simulink model "sim_2_twolink_joint_control_real"  (R2021a)
settings: Solver=ode45  StartTime=0.0  StopTime=15  MaxStep=0.01  RelTol=1e-5  EnableMultiTasking=on
values from neighbouring files (symbols this model uses):
  b1 = 0.01    [sim_params.m]    (also in sim_params_force.m)
  b2 = 0.01    [sim_params.m]    (also in sim_params_force.m)
  D = [zeros(n); eye(n)]    [control_comparison_script.m]    (also in gen_twolink_ss.m = reshape([0.0,0.0,0.0,0.0,0.0,0.0,0.0,0.0],[4,2]))
  D_T_Q = D'*Q    [control_comparison_script.m]
  epsilon = 0.1    [control_comparison_script.m]
  g = 9.80665    [sim_params.m]    (also in sim_params_force.m)
  joint_acc_variance = 0    [sim_params.m]    (also in sim_params_force.m)
  joint_pos_variance = joint_pos_precision^2    (= 0.0001)    [control_comparison_script.m]    (also in sim_params.m = 2.5e-05; sim_params_force.m = 2.5e-05)
  joint_vel_variance = 0    [sim_params.m]    (also in sim_params_force.m)
  Kd1 = 2.5    [control_comparison_script.m]
  Kd1_grav = 2.5    [control_comparison_script.m]
  Kd1_inv = 12    [control_comparison_script.m]
  Kd1_robust = 7    [control_comparison_script.m]
  Kd2 = 0.5    [control_comparison_script.m]
  Kd2_grav = 0.5    [control_comparison_script.m]
  Kd2_inv = 15    [control_comparison_script.m]
  Kd2_robust = 35    [control_comparison_script.m]
  Ki1 = 20    [control_comparison_script.m]
  Ki2 = 15    [control_comparison_script.m]
  Klqr = lqr(A,B,Q,R)    [control_comparison_script.m]
  Kp1 = 30    [control_comparison_script.m]
  Kp1_grav = 15    [control_comparison_script.m]
  Kp1_inv = 25    [control_comparison_script.m]
  Kp1_robust = 25    [control_comparison_script.m]
  Kp2 = 7    [control_comparison_script.m]
  Kp2_grav = 3.5    [control_comparison_script.m]
  Kp2_inv = 50    [control_comparison_script.m]
  Kp2_robust = 45    [control_comparison_script.m]
  Kpp = place(A,B,p)    [control_comparison_script.m]
  L1x = 0.3    [sim_params.m]    (also in sim_params_force.m)
  L1y = 0.050    (= 0.05)    [sim_params.m]    (also in sim_params_force.m)
  L1z = 0.05    [sim_params.m]    (also in sim_params_force.m)
  L2x = 0.15    [sim_params.m]    (also in sim_params_force.m = 0.3)
  L2y = 0.05    [sim_params.m]    (also in sim_params_force.m)
  L2z = 0.05    [sim_params.m]    (also in sim_params_force.m)
  length_dev = (100+randi([-param_dev,param_dev],1))/100.0    [control_comparison_script.m]
  m1 = m1*1.25    [control_comparison_script.m]    (also in sim_params.m = 2.775; sim_params_force.m = 2.775)
  m2 = m2*1.25    [control_comparison_script.m]    (also in sim_params.m = 1.3875; sim_params_force.m = 2.775)
  m_dev = (100+randi([-param_dev,param_dev],1))/100.0    [control_comparison_script.m]
  max_joint_torque1 = 20    [sim_params.m]    (also in sim_params_force.m)
  max_joint_torque2 = 10    [sim_params.m]    (also in sim_params_force.m = 20)
  N1 = 100    [control_comparison_script.m]
  N1_grav = 100    [control_comparison_script.m]
  N1_inv = 50    [control_comparison_script.m]
  N1_robust = 50    [control_comparison_script.m]
  N2 = 100    [control_comparison_script.m]
  N2_grav = 100    [control_comparison_script.m]
  N2_inv = 50    [control_comparison_script.m]
  N2_robust = 50    [control_comparison_script.m]
  rho = [1;1]    [control_comparison_script.m]
  theta1_0 = 0    [sim_params.m]    (also in sim_params_force.m = 1.57079632679)
  theta1_dot_0 = 0    [sim_params.m]    (also in sim_params_force.m)
  theta2_0 = 0    [sim_params.m]    (also in sim_params_force.m = -1.57079632679)
  theta2_dot_0 = 0    [sim_params.m]    (also in sim_params_force.m)
  Tsample = 0.001    [sim_params.m]    (also in sim_params_force.m)
  vis_dev = (100+randi([-param_dev,param_dev],1))/100.0    [control_comparison_script.m]
undefined symbols (not defined in the file or in its folder): gs, Ksm, phi_sm, sigbuilder_block, X, Y, Z
libraries: pid_lib x18, sm_lib x11, spsFirstOrderFilterLib x10, simulink_extras x10, nesl_utility x10, dspmtrx3 x2
(part 4 of 4)

== system sim_2_twolink_joint_control_real/Torqu limit/no-limit ==
  In1 : Inport
  Out1 : Outport
  wires:
  In1/1 -> Out1/1

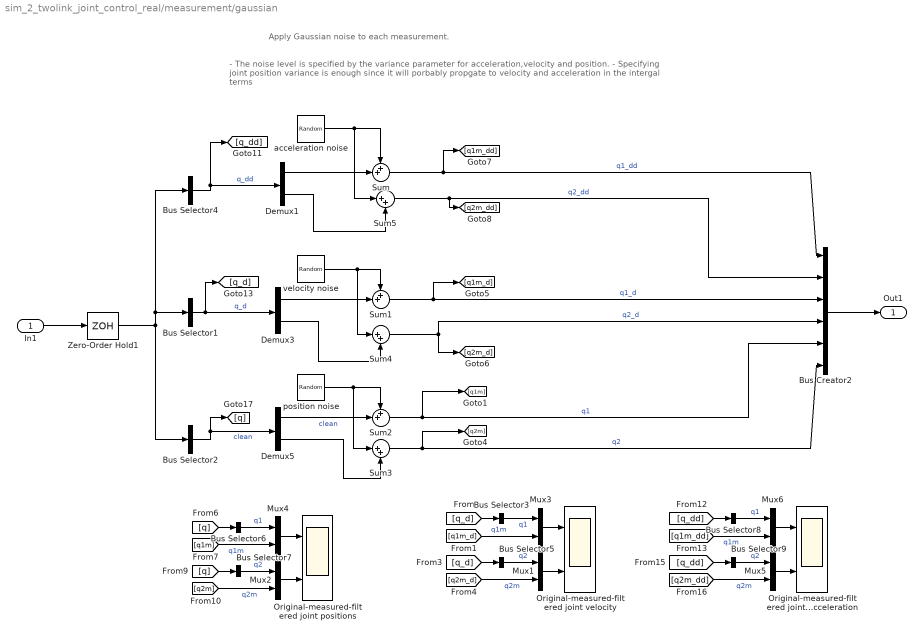
== system sim_2_twolink_joint_control_real/measurement/gaussian ==
  note: - The noise level is specified by the variance parameter for acceleration,velocity and position.
      | - Specifying joint position variance is enough since it will porbably propgate to velocity and acceleration in the intergal terms
  note: Apply Gaussian noise to each measurement.
  In1 : Inport
  Bus Creator2 : BusCreator  Inputs=6
  Bus Selector1 : BusSelector  OutputSignals=q1_d,q2_d  OutputAsBus=on
  Bus Selector2 : BusSelector  OutputSignals=q1,q2  OutputAsBus=on
  Bus Selector3 : BusSelector  OutputSignals=q1_d  OutputAsBus=on
  Bus Selector4 : BusSelector  OutputSignals=q1_dd,q2_dd  OutputAsBus=on
  Bus Selector5 : BusSelector  OutputSignals=q2_d  OutputAsBus=on
  Bus Selector6 : BusSelector  OutputSignals=q1  OutputAsBus=on
  Bus Selector7 : BusSelector  OutputSignals=q2  OutputAsBus=on
  Bus Selector8 : BusSelector  OutputSignals=q1_dd  OutputAsBus=on
  Bus Selector9 : BusSelector  OutputSignals=q2_dd  OutputAsBus=on
  Demux1 : Demux  Outputs=2
  Demux3 : Demux  Outputs=2
  Demux5 : Demux  Outputs=2
  Mux{1..6} (6 alike) : Mux  Inputs=2
  Original-measured-filtered joint Acceleration : Scope  NumInputPorts=2
  Original-measured-filtered joint positions : Scope  NumInputPorts=2
  Original-measured-filtered joint velocity : Scope  NumInputPorts=2
  Sum : Sum  Inputs=++|
  Sum1 : Sum  Inputs=++|
  Sum2 : Sum  Inputs=++|
  Sum3 : Sum  Inputs=|++
  Sum4 : Sum  Inputs=|++
  Sum5 : Sum  Inputs=|++
  Zero-Order Hold1 : ZeroOrderHold  SampleTime=Tsample
  acceleration noise : RandomNumber  Variance=joint_acc_variance  SampleTime=Tsample
  position noise : RandomNumber  Variance=joint_pos_variance  SampleTime=Tsample
  velocity noise : RandomNumber  Variance=joint_vel_variance  SampleTime=Tsample
  Out1 : Outport
  wires:
  In1/1 -> Zero-Order Hold1/1
  Demux1/1 -> Sum/2
  Demux3/2 -> Sum4/2
  Bus Selector3/1 -> Mux3/1  "q1"
  Mux2/1 -> Original-measured-filtered joint positions/2
  [q] -> Bus Selector6/1
  Bus Selector7/1 -> Mux2/1  "q2"
  [q1m] -> Mux4/2  "q1m"
  [q] -> Bus Selector7/1
  Bus Selector6/1 -> Mux4/1  "q1"
  Sum5/1 -> Bus Creator2/2, [q2m_dd]  "q2_dd"
  [q1m_d] -> Mux3/2  "q1m"
  Bus Selector4/1 -> [q_dd], Demux1/1  "q_dd"
  position noise/1 -> Sum2/1, Sum3/1
  Mux4/1 -> Original-measured-filtered joint positions/1
  velocity noise/1 -> Sum1/1, Sum4/1
  [q2m] -> Mux2/2  "q2m"
  Zero-Order Hold1/1 -> Bus Selector4/1, Bus Selector1/1, Bus Selector2/1
  Sum1/1 -> Bus Creator2/3, [q1m_d]  "q1_d"
  Mux5/1 -> Original-measured-filtered joint Acceleration/2
  Demux1/2 -> Sum5/2
  ? -> ?  "q2f"
  [q2m_dd] -> Mux5/2  "q2m"
  Bus Selector9/1 -> Mux5/1  "q2"
  [q_dd] -> Bus Selector8/1
  Sum2/1 -> Bus Creator2/5, [q1m]  "q1"
  acceleration noise/1 -> Sum5/1, Sum/1
  [q1m_dd] -> Mux6/2  "q1m"
  Bus Selector2/1 -> Demux5/1, [q]  "clean"
  Bus Creator2/1 -> Out1/1
  Bus Selector8/1 -> Mux6/1  "q1"
  [q_dd] -> Bus Selector9/1
  Mux6/1 -> Original-measured-filtered joint Acceleration/1
  Mux3/1 -> Original-measured-filtered joint velocity/1
  [q_d] -> Bus Selector3/1
  Demux5/1 -> Sum2/2  "clean"
  Demux5/2 -> Sum3/2
  Bus Selector5/1 -> Mux1/1  "q2"
  [q_d] -> Bus Selector5/1
  Bus Selector1/1 -> [q_d], Demux3/1  "q_d"
  Sum3/1 -> Bus Creator2/6, [q2m]  "q2"
  Sum/1 -> Bus Creator2/1, [q1m_dd]  "q1_dd"
  Sum4/1 -> Bus Creator2/4, [q2m_d]  "q2_d"
  [q2m_d] -> Mux1/2  "q2m"
  Demux3/1 -> Sum1/2
  Mux1/1 -> Original-measured-filtered joint velocity/2

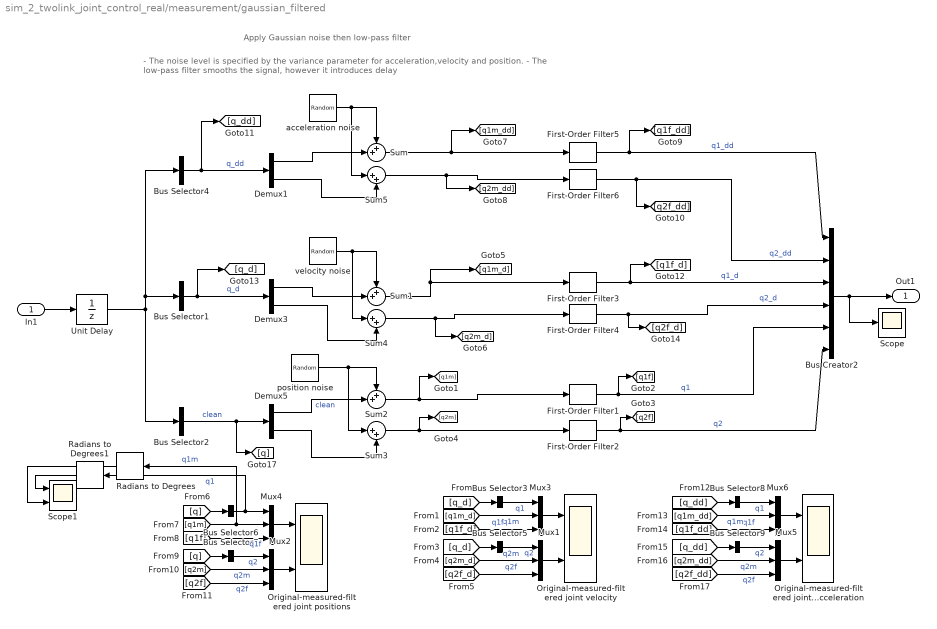
== system sim_2_twolink_joint_control_real/measurement/gaussian_filtered ==
  note: - The noise level is specified by the variance parameter for acceleration,velocity and position.
      | - The low-pass filter smooths the signal, however it introduces delay
  note: Apply Gaussian noise then low-pass filter
  In1 : Inport
  Bus Creator2 : BusCreator  Inputs=6
  Bus Selector1 : BusSelector  OutputSignals=q1_d,q2_d  OutputAsBus=on
  Bus Selector2 : BusSelector  OutputSignals=q1,q2  OutputAsBus=on
  Bus Selector3 : BusSelector  OutputSignals=q1_d  OutputAsBus=on
  Bus Selector4 : BusSelector  OutputSignals=q1_dd,q2_dd  OutputAsBus=on
  Bus Selector5 : BusSelector  OutputSignals=q2_d  OutputAsBus=on
  Bus Selector6 : BusSelector  OutputSignals=q1  OutputAsBus=on
  Bus Selector7 : BusSelector  OutputSignals=q2  OutputAsBus=on
  Bus Selector8 : BusSelector  OutputSignals=q1_dd  OutputAsBus=on
  Bus Selector9 : BusSelector  OutputSignals=q2_dd  OutputAsBus=on
  Demux1 : Demux  Outputs=2
  Demux3 : Demux  Outputs=2
  Demux5 : Demux  Outputs=2
  First-Order Filter1 : spsFirstOrderFilterLib/First-Order Filter  FilterType=Lowpass  Tc=0.006  Ts=Tsample  Initialize=on  Vac_Init=[0, 0, 0]  Vdc_Init=0  PlotResponse=off  FreqRange="[0,  200,  1]"
  First-Order Filter2 : spsFirstOrderFilterLib/First-Order Filter  FilterType=Lowpass  Tc=0.006  Ts=Tsample  Initialize=on  Vac_Init=[0, 0, 0]  Vdc_Init=0  PlotResponse=off  FreqRange="[0,  200,  1]"
  First-Order Filter3 : spsFirstOrderFilterLib/First-Order Filter  FilterType=Lowpass  Tc=0.05  Ts=Tsample  Initialize=on  Vac_Init=[0, 0, 0]  Vdc_Init=0  PlotResponse=off  FreqRange="[0,  200,  1]"
  First-Order Filter4 : spsFirstOrderFilterLib/First-Order Filter  FilterType=Lowpass  Tc=0.05  Ts=Tsample  Initialize=on  Vac_Init=[0, 0, 0]  Vdc_Init=0  PlotResponse=off  FreqRange="[0,  200,  1]"
  First-Order Filter5 : spsFirstOrderFilterLib/First-Order Filter  FilterType=Lowpass  Tc=0.1  Ts=Tsample  Initialize=on  Vac_Init=[0, 0, 0]  Vdc_Init=0  PlotResponse=off  FreqRange="[0,  200,  1]"
  First-Order Filter6 : spsFirstOrderFilterLib/First-Order Filter  FilterType=Lowpass  Tc=0.1  Ts=Tsample  Initialize=on  Vac_Init=[0, 0, 0]  Vdc_Init=0  PlotResponse=off  FreqRange="[0,  200,  1]"
  Mux{1..6} (6 alike) : Mux  Inputs=3
  Original-measured-filtered joint Acceleration : Scope  NumInputPorts=2
  Original-measured-filtered joint positions : Scope  NumInputPorts=2
  Original-measured-filtered joint velocity : Scope  NumInputPorts=2
  Radians to Degrees : simulink_extras/Transformations/Radians to Degrees
  Radians to Degrees1 : simulink_extras/Transformations/Radians to Degrees
  Scope : Scope
  Scope1 : Scope  NumInputPorts=2
  Sum : Sum  Inputs=++|
  Sum1 : Sum  Inputs=++|
  Sum2 : Sum  Inputs=++|
  Sum3 : Sum  Inputs=|++
  Sum4 : Sum  Inputs=|++
  Sum5 : Sum  Inputs=|++
  Unit Delay : UnitDelay  SampleTime=Tsample  HasFrameUpgradeWarning=on
  acceleration noise : RandomNumber  Variance=joint_acc_variance  SampleTime=Tsample
  position noise : RandomNumber  Variance=joint_pos_variance  SampleTime=Tsample
  velocity noise : RandomNumber  Variance=joint_vel_variance  SampleTime=Tsample
  Out1 : Outport
  wires:
  acceleration noise/1 -> Sum/1, Sum5/1
  Bus Selector4/1 -> [q_dd], Demux1/1  "q_dd"
  Sum4/1 -> First-Order Filter4/1, [q2m_d]
  velocity noise/1 -> Sum1/1, Sum4/1
  Demux3/1 -> Sum1/2
  Bus Selector1/1 -> [q_d], Demux3/1  "q_d"
  Sum2/1 -> [q1m], First-Order Filter1/1
  position noise/1 -> Sum2/1, Sum3/1
  Demux5/1 -> Sum2/2  "clean"
  In1/1 -> Unit Delay/1
  Bus Creator2/1 -> Scope/1, Out1/1
  First-Order Filter2/1 -> Bus Creator2/6, [q2f]  "q2"
  First-Order Filter1/1 -> Bus Creator2/5, [q1f]  "q1"
  First-Order Filter3/1 -> Bus Creator2/3, [q1f_d]  "q1_d"
  First-Order Filter4/1 -> Bus Creator2/4, [q2f_d]  "q2_d"
  First-Order Filter6/1 -> Bus Creator2/2, [q2f_dd]  "q2_dd"
  [q_d] -> Bus Selector3/1
  Mux3/1 -> Original-measured-filtered joint velocity/1
  Bus Selector3/1 -> Mux3/1  "q1"
  Bus Selector2/1 -> [q], Demux5/1  "clean"
  Demux5/2 -> Sum3/2
  Sum3/1 -> [q2m], First-Order Filter2/1
  [q1m_d] -> Mux3/2  "q1m"
  [q1f_d] -> Mux3/3  "q1f"
  [q2m_d] -> Mux1/2  "q2m"
  Mux1/1 -> Original-measured-filtered joint velocity/2
  [q2f_d] -> Mux1/3  "q2f"
  Bus Selector5/1 -> Mux1/1  "q2"
  [q_d] -> Bus Selector5/1
  Demux3/2 -> Sum4/2
  Sum1/1 -> First-Order Filter3/1, [q1m_d]
  Demux1/1 -> Sum/2
  Demux1/2 -> Sum5/2
  Sum/1 -> [q1m_dd], First-Order Filter5/1
  Sum5/1 -> [q2m_dd], First-Order Filter6/1
  Bus Selector6/1 -> Radians to Degrees1/1, Mux4/1  "q1"
  [q1f] -> Mux4/3  "q1f"
  [q1m] -> Radians to Degrees/1, Mux4/2  "q1m"
  Mux4/1 -> Original-measured-filtered joint positions/1
  Bus Selector7/1 -> Mux2/1  "q2"
  [q] -> Bus Selector7/1
  [q2m] -> Mux2/2  "q2m"
  [q] -> Bus Selector6/1
  Mux2/1 -> Original-measured-filtered joint positions/2
  [q2f] -> Mux2/3  "q2f"
  Bus Selector8/1 -> Mux6/1  "q1"
  [q1f_dd] -> Mux6/3  "q1f"
  [q1m_dd] -> Mux6/2  "q1m"
  Mux6/1 -> Original-measured-filtered joint Acceleration/1
  Bus Selector9/1 -> Mux5/1  "q2"
  [q_dd] -> Bus Selector9/1
  [q2m_dd] -> Mux5/2  "q2m"
  [q_dd] -> Bus Selector8/1
  Mux5/1 -> Original-measured-filtered joint Acceleration/2
  [q2f_dd] -> Mux5/3  "q2f"
  First-Order Filter5/1 -> Bus Creator2/1, [q1f_dd]  "q1_dd"
  Unit Delay/1 -> Bus Selector4/1, Bus Selector1/1, Bus Selector2/1
  Radians to Degrees1/1 -> Scope1/1
  Radians to Degrees/1 -> Scope1/2

== system sim_2_twolink_joint_control_real/measurement/ideal ==
  In1 : Inport
  Zero-Order Hold1 : ZeroOrderHold  SampleTime=Tsample
  Out1 : Outport
  wires:
  In1/1 -> Zero-Order Hold1/1
  Zero-Order Hold1/1 -> Out1/1

== system sim_2_twolink_joint_control_real/Commands/Step command/Joint commands ==
  Demux : Demux  Tag=STV Demux  Outputs=2
      settings: DisplayOption=none
  FromWs : FromWorkspace  Tag=STV FromWs  VariableName=tuvar
      SigBuilderData=|
      | common.afterFinalStr = 'Extrapolate'
      | common.sampleTime = 0
      | dataSet(1).timeRange = [0 1000]
      | dataSet(1).name = 'PULSES_SMALL'
      | dataSet(2).timeRange = [0 1000]
      | dataSet(2).name = 'ZERO'
      | dataSet(3).timeRange = [0 1000]
      | dataSet(3).name = 'PULSES_BIG'
      | dataSet(4).timeRange = [0 1000]
      | dataSet(4).name = 'PULSES_SMALL1'
      | sbobj.Groups(1).Name = 'PULSES_SMALL'
      | sbobj.Groups(1).Signals(1).Name = 'cmd_q1'
      | sbobj.Groups(1).Signals(1).XData = [0 5 5 11 11 15 15 1000]
      | sbobj.Groups(1).Signals(1).YData = [0 0 1.5 1.5 0.7 0.7 0 0]
      | sbobj.Groups(1).Signals(2).Name = 'cmd_q2'
      | sbobj.Groups(1).Signals(2).XData = [0 4 4 8 8 15 15 1000]
      | sbobj.Groups(1).Signals(2).YData = [0 0 0.5 0.5 1 1 0 0]
      | sbobj.Groups(1).TimeRange = [0 1000]
      | sbobj.Groups(2).Name = 'ZERO'
      | sbobj.Groups(2).Signals(1).Name = 'cmd_q1'
      | sbobj.Groups(2).Signals(1).XData = [0 500 500 1000]
      | sbobj.Groups(2).Signals(1).YData = [0 0 1 1]
      | sbobj.Groups(2).Signals(2).Name = 'cmd_q2'
      | sbobj.Groups(2).Signals(2).XData = [0 1000]
      | sbobj.Groups(2).Signals(2).YData = [0 0]
      | sbobj.Groups(2).TimeRange = [0 1000]
      | sbobj.Groups(3).Name = 'PULSES_BIG'
      | sbobj.Groups(3).Signals(1).Name = 'cmd_q1'
      | sbobj.Groups(3).Signals(1).XData = [0 500 500 1000]
      | sbobj.Groups(3).Signals(1).YData = [0 0 1 1]
      | sbobj.Groups(3).Signals(2).Name = 'cmd_q2'
      | sbobj.Groups(3).Signals(2).XData = [0 1000]
      | sbobj.Groups(3).Signals(2).YData = [0 0]
      | sbobj.Groups(3).TimeRange = [0 1000]
      | sbobj.Groups(4).Name = 'PULSES_SMALL1'
      | sbobj.Groups(4).Signals(1).Name = 'cmd_q1'
      | sbobj.Groups(4).Signals(1).XData = [0 500 500 1000]
      | sbobj.Groups(4).Signals(1).YData = [0 0 1 1]
      | sbobj.Groups(4).Signals(2).Name = 'cmd_q2'
      | sbobj.Groups(4).Signals(2).XData = [0 1000]
      | sbobj.Groups(4).Signals(2).YData = [0 0]
      | sbobj.Groups(4).TimeRange = [0 1000]
  cmd_q1 : Outport  Tag=STV Outport
  cmd_q2 : Outport  Tag=STV Outport  Port=2
  wires:
  FromWs/1 -> Demux/1
  Demux/1 -> cmd_q1/1
  Demux/2 -> cmd_q2/1

== system sim_2_twolink_joint_control_real/Commands/Trapezoidal velocity/Joint commands ==
  Demux : Demux  Tag=STV Demux  Outputs=2
      settings: DisplayOption=none
  FromWs : FromWorkspace  Tag=STV FromWs  VariableName=tuvar
      SigBuilderData=|
      | common.afterFinalStr = 'Extrapolate'
      | common.sampleTime = 0
      | dataSet(1).timeRange = [0 1000]
      | dataSet(1).name = 'PULSES_SMALL'
      | dataSet(2).timeRange = [0 1000]
      | dataSet(2).name = 'ZERO'
      | dataSet(3).timeRange = [0 1000]
      | dataSet(3).name = 'PULSES_BIG'
      | dataSet(4).timeRange = [0 1000]
      | dataSet(4).name = 'PULSES_SMALL1'
      | sbobj.Groups(1).Name = 'PULSES_SMALL'
      | sbobj.Groups(1).Signals(1).Name = 'cmd_q1_dot'
      | sbobj.Groups(1).Signals(1).XData = [0 2 4 6 8 10 12 14 1000]
      | sbobj.Groups(1).Signals(1).YData = [0 0 0 0 0.4 0.4 0 0 0]
      | sbobj.Groups(1).Signals(2).Name = 'cmd_q2_dot'
      | sbobj.Groups(1).Signals(2).XData = [0 2 4 6 8 10 1000]
      | sbobj.Groups(1).Signals(2).YData = [0 0 0.4 0.4 0 0 0]
      | sbobj.Groups(1).TimeRange = [0 1000]
      | sbobj.Groups(2).Name = 'ZERO'
      | sbobj.Groups(2).Signals(1).Name = 'cmd_q1_dot'
      | sbobj.Groups(2).Signals(1).XData = [0 5 10 15 1000]
      | sbobj.Groups(2).Signals(1).YData = [0 1 1 0 0]
      | sbobj.Groups(2).Signals(2).Name = 'cmd_q2_dot'
      | sbobj.Groups(2).Signals(2).XData = [0 5 10 15 1000]
      | sbobj.Groups(2).Signals(2).YData = [0 1 1 0 0]
      | sbobj.Groups(2).TimeRange = [0 1000]
      | sbobj.Groups(3).Name = 'PULSES_BIG'
      | sbobj.Groups(3).Signals(1).Name = 'cmd_q1_dot'
      | sbobj.Groups(3).Signals(1).XData = [0 5 10 15 1000]
      | sbobj.Groups(3).Signals(1).YData = [0 1 1 0 0]
      | sbobj.Groups(3).Signals(2).Name = 'cmd_q2_dot'
      | sbobj.Groups(3).Signals(2).XData = [0 5 10 15 1000]
      | sbobj.Groups(3).Signals(2).YData = [0 1 1 0 0]
      | sbobj.Groups(3).TimeRange = [0 1000]
      | sbobj.Groups(4).Name = 'PULSES_SMALL1'
      | sbobj.Groups(4).Signals(1).Name = 'cmd_q1_dot'
      | sbobj.Groups(4).Signals(1).XData = [0 5 10 15 1000]
      | sbobj.Groups(4).Signals(1).YData = [0 1 1 0 0]
      | sbobj.Groups(4).Signals(2).Name = 'cmd_q2_dot'
      | sbobj.Groups(4).Signals(2).XData = [0 5 10 15 1000]
      | sbobj.Groups(4).Signals(2).YData = [0 1 1 0 0]
      | sbobj.Groups(4).TimeRange = [0 1000]
  cmd_q1_dot : Outport  Tag=STV Outport
  cmd_q2_dot : Outport  Tag=STV Outport  Port=2
  wires:
  FromWs/1 -> Demux/1
  Demux/1 -> cmd_q1_dot/1
  Demux/2 -> cmd_q2_dot/1

== system sim_2_twolink_joint_control_real/Controller/Inverse Dynamics PID control /FeedForward terms ==
  C : Inport
  K : Inport  Port=2
  G : Inport  Port=3
  q : Inport  Port=4
  q_d : Inport  Port=5
  q_dd : Inport  Port=6
  M : Inport  Port=7
  F : Inport  Port=8
  Product : Product  Multiplication=Matrix(*)
  Product2 : Product  Multiplication=Matrix(*)
  Product3 : Product  Multiplication=Matrix(*)
  Sum : Sum  Inputs=+|+|+|+
  Terminator : Terminator
  Q : Outport
  wires:
  K/1 -> Product/1
  Product/1 -> Sum/3
  Product2/1 -> Sum/1
  Sum/1 -> Q/1
  C/1 -> Product3/1
  Product3/1 -> Sum/2
  M/1 -> Product2/1
  q_dd/1 -> Product2/2
  q/1 -> Product/2
  q_d/1 -> Product3/2
  F/1 -> Terminator/1
  G/1 -> Sum/4

== system sim_2_twolink_joint_control_real/Controller/Inverse Dynamics control /FeedForward terms ==
  C : Inport
  K : Inport  Port=2
  G : Inport  Port=3
  q : Inport  Port=4
  q_d : Inport  Port=5
  q_dd : Inport  Port=6
  M : Inport  Port=7
  F : Inport  Port=8
  Product : Product  Multiplication=Matrix(*)
  Product2 : Product  Multiplication=Matrix(*)
  Product3 : Product  Multiplication=Matrix(*)
  Sum : Sum  Inputs=+|+|+|+
  Terminator : Terminator
  Q : Outport
  wires:
  K/1 -> Product/1
  Product/1 -> Sum/3
  Product2/1 -> Sum/1
  Sum/1 -> Q/1
  C/1 -> Product3/1
  Product3/1 -> Sum/2
  M/1 -> Product2/1
  q_dd/1 -> Product2/2
  q/1 -> Product/2
  q_d/1 -> Product3/2
  F/1 -> Terminator/1
  G/1 -> Sum/4

== matlab function sim_2_twolink_joint_control_real/Controller/Robust control /Gravity compensation ==
  data: L_1x input; G output; L_2x input; g input; m1 input; m2 input; q1 input; q2 input
function G = G_compensation(L_1x,L_2x,g,m1,m2,q1,q2)
%#codegen

%    This function was generated by the Symbolic Math Toolbox version 8.7.
%    01-Jun-2022 14:38:05

G = [(g.*(L_2x.*m2.*cos(q1+q2)+L_1x.*m1.*cos(q1)+L_1x.*m2.*cos(q1).*2.0))./2.0;
    (L_2x.*g.*m2.*cos(q1+q2))./2.0];

== matlab function sim_2_twolink_joint_control_real/Controller/PD-gravity Control /Gravity compensation ==
  data: L_1x input; G output; L_2x input; g input; m1 input; m2 input; q1 input; q2 input
function G = G_compensation(L_1x,L_2x,g,m1,m2,q1,q2)
%#codegen

%    This function was generated by the Symbolic Math Toolbox version 8.7.
%    01-Jun-2022 14:38:05

G = [(g.*(L_2x.*m2.*cos(q1+q2)+L_1x.*m1.*cos(q1)+L_1x.*m2.*cos(q1).*2.0))./2.0;(L_2x.*g.*m2.*cos(q1+q2))./2.0];

== matlab function sim_2_twolink_joint_control_real/Controller/Robust control /MATLAB Function ==
  data: z input; w output; epsilon input; rho input
function w = fcn(z, epsilon, rho)
    z_norm = norm(z);
    if z_norm>=epsilon
        w = (rho/z_norm).*z;
    else
        w = (rho/epsilon).*z;
    end

== matlab function sim_2_twolink_joint_control_real/Controller/Inverse Dynamics PID control /MCKGQ ==
  data: L_1x input; M output; L_1y input; L_2x input; L_2y input; b1 input; b2 input; g input; m1 input; m2 input; q1 input; q2 input; q1_D input; q2_D input; tau1 input; tau2 input; C output; K output; G output; Q output
function [M,C,K,G,Q] = MCKGQ(L_1x,L_1y,L_2x,L_2y,b1,b2,g,m1,m2,q1,q2,q1_D,q2_D,tau1,tau2)
%#codegen

%    This function was generated by the Symbolic Math Toolbox version 8.7.
%    30-May-2022 13:59:37

M = reshape([(L_1x.^2.*m1)./3.0+L_1x.^2.*m2+(L_1y.^2.*m1)./1.2e+1+(L_2x.^2.*m2)./4.0+L_1x.*L_2x.*m2.*cos(q2),(L_2x.*m2.*(L_2x+L_1x.*cos(q2).*2.0))./4.0,(L_2x.*m2.*(L_2x+L_1x.*cos(q2).*2.0))./4.0,(m2.*(L_2x.^2.*4.0+L_2y.^2))./1.2e+1],[2,2]);
if nargout > 1
    C = reshape([-L_1x.*L_2x.*m2.*q2_D.*sin(q2),(L_1x.*L_2x.*m2.*q1_D.*sin(q2))./2.0,L_1x.*L_2x.*m2.*q2_D.*sin(q2).*(-1.0./2.0),0.0],[2,2]);
end
if nargout > 2
    K = reshape([0.0,0.0,0.0,0.0],[2,2]);
end
if nargout > 3
    G = [(g.*(L_2x.*m2.*cos(q1+q2)+L_1x.*m1.*cos(q1)+L_1x.*m2.*cos(q1).*2.0))./2.0;(L_2x.*g.*m2.*cos(q1+q2))./2.0];
end
if nargout > 4
    Q = [tau1-b1.*q1_D;tau2-b2.*q2_D];
end

== matlab function sim_2_twolink_joint_control_real/Controller/Robust control /simplified_model ==
  data: L_1x input; M_bar output; L_1y input; L_2x input; L_2y input; b1 input; b2 input; m1 input; m2 input; Fv output
function [M_bar,Fv] = simplified_model(L_1x,L_1y,L_2x,L_2y,b1,b2,m1,m2)
%#codegen

%    This function was generated by the Symbolic Math Toolbox version 8.7.
%    17-Jun-2022 16:27:20

M_bar = reshape([(L_1x.^2.*m1)./3.0+L_1x.^2.*m2+(L_1y.^2.*m1)./1.2e+1+(L_2x.^2.*m2)./4.0,0.0,0.0,(m2.*(L_2x.^2.*4.0+L_2y.^2))./1.2e+1],[2,2]);
if nargout > 1
    Fv = reshape([b1,0.0,0.0,b2],[2,2]);
end

== matlab function sim_2_twolink_joint_control_real/Controller/Robust PID control /Gravity compensation ==
  data: L_1x input; G output; L_2x input; g input; m1 input; m2 input; q1 input; q2 input
function G = G_compensation(L_1x,L_2x,g,m1,m2,q1,q2)
%#codegen

%    This function was generated by the Symbolic Math Toolbox version 8.7.
%    01-Jun-2022 14:38:05

G = [(g.*(L_2x.*m2.*cos(q1+q2)+L_1x.*m1.*cos(q1)+L_1x.*m2.*cos(q1).*2.0))./2.0;
    (L_2x.*g.*m2.*cos(q1+q2))./2.0];

== matlab function sim_2_twolink_joint_control_real/Controller/Robust PID control /MATLAB Function ==
  data: z input; w output; epsilon input; rho input
function w = fcn(z, epsilon, rho)
    z_norm = norm(z);
    if z_norm>=epsilon
        w = (rho/z_norm).*z;
    else
        w = (rho/epsilon).*z;
    end

== matlab function sim_2_twolink_joint_control_real/Controller/Robust PID control /simplified_model ==
  data: L_1x input; M_bar output; L_1y input; L_2x input; L_2y input; b1 input; b2 input; m1 input; m2 input; Fv output
function [M_bar,Fv] = simplified_model(L_1x,L_1y,L_2x,L_2y,b1,b2,m1,m2)
%#codegen

%    This function was generated by the Symbolic Math Toolbox version 8.7.
%    17-Jun-2022 16:27:20

M_bar = reshape([(L_1x.^2.*m1)./3.0+L_1x.^2.*m2+(L_1y.^2.*m1)./1.2e+1+(L_2x.^2.*m2)./4.0,0.0,0.0,(m2.*(L_2x.^2.*4.0+L_2y.^2))./1.2e+1],[2,2]);
if nargout > 1
    Fv = reshape([b1,0.0,0.0,b2],[2,2]);
end

== matlab function sim_2_twolink_joint_control_real/Controller/PID-gravity Control/Gravity compensation ==
  data: L_1x input; G output; L_2x input; g input; m1 input; m2 input; q1 input; q2 input
function G = G_compensation(L_1x,L_2x,g,m1,m2,q1,q2)
%#codegen

%    This function was generated by the Symbolic Math Toolbox version 8.7.
%    01-Jun-2022 14:38:05

G = [(g.*(L_2x.*m2.*cos(q1+q2)+L_1x.*m1.*cos(q1)+L_1x.*m2.*cos(q1).*2.0))./2.0;(L_2x.*g.*m2.*cos(q1+q2))./2.0];

== matlab function sim_2_twolink_joint_control_real/Controller/LQR+D Control/disturbance_terms ==
  data: L_1x input; d output; L_2x input; g input; m1 input; m2 input; q1 input; q2 input; q1_D input; q2_D input; q1_DD input; q2_DD input
function d = disturbance_terms(L_1x,L_2x,g,m1,m2,q1,q2,q1_D,q2_D,q1_DD,q2_DD)
%#codegen

%    This function was generated by the Symbolic Math Toolbox version 8.7.
%    10-Jun-2022 15:47:18

d = [(g.*(L_2x.*m2.*cos(q1+q2)+L_1x.*m1.*cos(q1)+L_1x.*m2.*cos(q1).*2.0))./2.0+(L_2x.*m2.*q2_DD.*(L_2x+L_1x.*cos(q2).*2.0))./4.0-(L_1x.*L_2x.*m2.*q2_D.^2.*sin(q2))./2.0+L_1x.*L_2x.*m2.*q1_DD.*cos(q2)-L_1x.*L_2x.*m2.*q1_D.*q2_D.*sin(q2);(L_2x.*g.*m2.*cos(q1+q2))./2.0+(L_2x.*m2.*q1_DD.*(L_2x+L_1x.*cos(q2).*2.0))./4.0+(L_1x.*L_2x.*m2.*q1_D.^2.*sin(q2))./2.0];

== matlab function sim_2_twolink_joint_control_real/Robot/SIMULINK_MODEL/THE_TH_DD ==
  data: L_1x input; theta_DD output; L_1y input; L_2x input; L_2y input; b1 input; b2 input; g input; m1 input; m2 input; q1 input; q2 input; q1_D input; q2_D input; tau1 input; tau2 input
function theta_DD = THE_TH_DD(L_1x,L_1y,L_2x,L_2y,b1,b2,g,m1,m2,q1,q2,q1_D,q2_D,tau1,tau2)
%#codegen

%    This function was generated by the Symbolic Math Toolbox version 8.7.
%    30-May-2022 13:59:37

et1 = (L_1x.^2.*m1.*4.0+L_1x.^2.*m2.*1.2e+1+L_1y.^2.*m1+L_2x.^2.*m2.*3.0+L_1x.*L_2x.*m2.*cos(q2).*1.2e+1).*(-tau2+b2.*q2_D+(L_1x.*L_2x.*m2.*q1_D.^2.*sin(q2))./2.0+(L_2x.*g.*m2.*cos(q1).*cos(q2))./2.0-(L_2x.*g.*m2.*sin(q1).*sin(q2))./2.0);
et2 = -1.2e+1./(L_2x.^4.*m2.^2.*3.0+L_1x.^2.*L_2x.^2.*m2.^2.*4.8e+1+L_1x.^2.*L_2y.^2.*m2.^2.*1.2e+1+L_2x.^2.*L_2y.^2.*m2.^2.*3.0+L_1x.^2.*L_2x.^2.*m1.*m2.*1.6e+1+L_1x.^2.*L_2y.^2.*m1.*m2.*4.0+L_1y.^2.*L_2x.^2.*m1.*m2.*4.0+L_1y.^2.*L_2y.^2.*m1.*m2-L_1x.^2.*L_2x.^2.*m2.^2.*cos(q2).^2.*3.6e+1+L_1x.*L_2x.^3.*m2.^2.*cos(q2).*1.2e+1+L_1x.*L_2x.*L_2y.^2.*m2.^2.*cos(q2).*1.2e+1);
et3 = ((L_2x.^2+L_1x.*L_2x.*cos(q2).*2.0).*(-tau2+b2.*q2_D+(L_1x.*L_2x.*m2.*q1_D.^2.*sin(q2))./2.0+(L_2x.*g.*m2.*cos(q1).*cos(q2))./2.0-(L_2x.*g.*m2.*sin(q1).*sin(q2))./2.0).*3.6e+1)./(L_2x.^4.*m2.*3.0+L_1x.^2.*L_2x.^2.*m1.*1.6e+1+L_1x.^2.*L_2x.^2.*m2.*4.8e+1+L_1x.^2.*L_2y.^2.*m1.*4.0+L_1y.^2.*L_2x.^2.*m1.*4.0+L_1x.^2.*L_2y.^2.*m2.*1.2e+1+L_1y.^2.*L_2y.^2.*m1+L_2x.^2.*L_2y.^2.*m2.*3.0-L_1x.^2.*L_2x.^2.*m2.*cos(q2).^2.*3.6e+1+L_1x.*L_2x.^3.*m2.*cos(q2).*1.2e+1+L_1x.*L_2x.*L_2y.^2.*m2.*cos(q2).*1.2e+1);
et4 = ((L_2x.^2.*4.0+L_2y.^2).*(tau1-b1.*q1_D-(L_1x.*g.*m1.*cos(q1))./2.0-L_1x.*g.*m2.*cos(q1)+(L_1x.*L_2x.*m2.*q2_D.^2.*sin(q2))./2.0-(L_2x.*g.*m2.*cos(q1).*cos(q2))./2.0+(L_2x.*g.*m2.*sin(q1).*sin(q2))./2.0+L_1x.*L_2x.*m2.*q1_D.*q2_D.*sin(q2)).*1.2e+1)./(L_2x.^4.*m2.*3.0+L_1x.^2.*L_2x.^2.*m1.*1.6e+1+L_1x.^2.*L_2x.^2.*m2.*4.8e+1+L_1x.^2.*L_2y.^2.*m1.*4.0+L_1y.^2.*L_2x.^2.*m1.*4.0+L_1x.^2.*L_2y.^2.*m2.*1.2e+1+L_1y.^2.*L_2y.^2.*m1+L_2x.^2.*L_2y.^2.*m2.*3.0-L_1x.^2.*L_2x.^2.*m2.*cos(q2).^2.*3.6e+1+L_1x.*L_2x.^3.*m2.*cos(q2).*1.2e+1+L_1x.*L_2x.*L_2y.^2.*m2.*cos(q2).*1.2e+1);
theta_DD = [et3+et4;et1.*et2-((L_2x.^2+L_1x.*L_2x.*cos(q2).*2.0).*(tau1-b1.*q1_D-(L_1x.*g.*m1.*cos(q1))./2.0-L_1x.*g.*m2.*cos(q1)+(L_1x.*L_2x.*m2.*q2_D.^2.*sin(q2))./2.0-(L_2x.*g.*m2.*cos(q1).*cos(q2))./2.0+(L_2x.*g.*m2.*sin(q1).*sin(q2))./2.0+L_1x.*L_2x.*m2.*q1_D.*q2_D.*sin(q2)).*3.6e+1)./(L_2x.^4.*m2.*3.0+L_1x.^2.*L_2x.^2.*m1.*1.6e+1+L_1x.^2.*L_2x.^2.*m2.*4.8e+1+L_1x.^2.*L_2y.^2.*m1.*4.0+L_1y.^2.*L_2x.^2.*m1.*4.0+L_1x.^2.*L_2y.^2.*m2.*1.2e+1+L_1y.^2.*L_2y.^2.*m1+L_2x.^2.*L_2y.^2.*m2.*3.0-L_1x.^2.*L_2x.^2.*m2.*cos(q2).^2.*3.6e+1+L_1x.*L_2x.^3.*m2.*cos(q2).*1.2e+1+L_1x.*L_2x.*L_2y.^2.*m2.*cos(q2).*1.2e+1)];

== matlab function sim_2_twolink_joint_control_real/Controller/Robust LQR+D Control/disturbance_terms ==
  data: L_1x input; d output; L_2x input; g input; m1 input; m2 input; q1 input; q2 input; q1_D input; q2_D input; q1_DD input; q2_DD input
function d = disturbance_terms(L_1x,L_2x,g,m1,m2,q1,q2,q1_D,q2_D,q1_DD,q2_DD)
%#codegen

%    This function was generated by the Symbolic Math Toolbox version 8.7.
%    10-Jun-2022 15:47:18

d = [(g.*(L_2x.*m2.*cos(q1+q2)+L_1x.*m1.*cos(q1)+L_1x.*m2.*cos(q1).*2.0))./2.0+(L_2x.*m2.*q2_DD.*(L_2x+L_1x.*cos(q2).*2.0))./4.0-(L_1x.*L_2x.*m2.*q2_D.^2.*sin(q2))./2.0+L_1x.*L_2x.*m2.*q1_DD.*cos(q2)-L_1x.*L_2x.*m2.*q1_D.*q2_D.*sin(q2);(L_2x.*g.*m2.*cos(q1+q2))./2.0+(L_2x.*m2.*q1_DD.*(L_2x+L_1x.*cos(q2).*2.0))./4.0+(L_1x.*L_2x.*m2.*q1_D.^2.*sin(q2))./2.0];

== matlab function sim_2_twolink_joint_control_real/Controller/Robust LQR+D Control/MATLAB Function ==
  data: S input; w output; phi input
function w = sat_sm(S, phi)
    w = sign(S);
    if abs(S(1))<=phi(1)
        w(1) = S(1)/phi(1);
    end
    if abs(S(2))<=phi(2)
        w(2) = S(2)/phi(2);
    end

== matlab function sim_2_twolink_joint_control_real/Controller/Pole Placement+D Control/disturbance_terms ==
  data: L_1x input; d output; L_2x input; g input; m1 input; m2 input; q1 input; q2 input; q1_D input; q2_D input; q1_DD input; q2_DD input
function d = disturbance_terms(L_1x,L_2x,g,m1,m2,q1,q2,q1_D,q2_D,q1_DD,q2_DD)
%#codegen

%    This function was generated by the Symbolic Math Toolbox version 8.7.
%    10-Jun-2022 15:47:18

d = [(g.*(L_2x.*m2.*cos(q1+q2)+L_1x.*m1.*cos(q1)+L_1x.*m2.*cos(q1).*2.0))./2.0+(L_2x.*m2.*q2_DD.*(L_2x+L_1x.*cos(q2).*2.0))./4.0-(L_1x.*L_2x.*m2.*q2_D.^2.*sin(q2))./2.0+L_1x.*L_2x.*m2.*q1_DD.*cos(q2)-L_1x.*L_2x.*m2.*q1_D.*q2_D.*sin(q2);(L_2x.*g.*m2.*cos(q1+q2))./2.0+(L_2x.*m2.*q1_DD.*(L_2x+L_1x.*cos(q2).*2.0))./4.0+(L_1x.*L_2x.*m2.*q1_D.^2.*sin(q2))./2.0];

== matlab function sim_2_twolink_joint_control_real/Robot/SIMULINK_MODEL/MCKGQ ==
  data: L_1x input; M output; L_1y input; L_2x input; L_2y input; b1 input; b2 input; g input; m1 input; m2 input; q1 input; q2 input; q1_D input; q2_D input; tau1 input; tau2 input; C output; K output; G output; Q output
function [M,C,K,G,Q] = MCKGQ(L_1x,L_1y,L_2x,L_2y,b1,b2,g,m1,m2,q1,q2,q1_D,q2_D,tau1,tau2)
%#codegen

%    This function was generated by the Symbolic Math Toolbox version 8.7.
%    30-May-2022 13:59:37

M = reshape([(L_1x.^2.*m1)./3.0+L_1x.^2.*m2+(L_1y.^2.*m1)./1.2e+1+(L_2x.^2.*m2)./4.0+L_1x.*L_2x.*m2.*cos(q2),(L_2x.*m2.*(L_2x+L_1x.*cos(q2).*2.0))./4.0,(L_2x.*m2.*(L_2x+L_1x.*cos(q2).*2.0))./4.0,(m2.*(L_2x.^2.*4.0+L_2y.^2))./1.2e+1],[2,2]);
if nargout > 1
    C = reshape([-L_1x.*L_2x.*m2.*q2_D.*sin(q2),(L_1x.*L_2x.*m2.*q1_D.*sin(q2))./2.0,L_1x.*L_2x.*m2.*q2_D.*sin(q2).*(-1.0./2.0),0.0],[2,2]);
end
if nargout > 2
    K = reshape([0.0,0.0,0.0,0.0],[2,2]);
end
if nargout > 3
    G = [(g.*(L_2x.*m2.*cos(q1+q2)+L_1x.*m1.*cos(q1)+L_1x.*m2.*cos(q1).*2.0))./2.0;(L_2x.*g.*m2.*cos(q1+q2))./2.0];
end
if nargout > 4
    Q = [tau1-b1.*q1_D;tau2-b2.*q2_D];
end

== matlab function sim_2_twolink_joint_control_real/Robot/SIMULINK_MODEL/MATLAB Function1 ==
  data: M input; the_cond output
function the_cond = COND(M)
%#codegen

the_cond = cond(M);

end

== matlab function sim_2_twolink_joint_control_real/Controller/PD_plus_gravity_plus_feadforward/Gravity compensation ==
  data: L_1x input; G output; L_2x input; g input; m1 input; m2 input; q1 input; q2 input
function G = G_compensation(L_1x,L_2x,g,m1,m2,q1,q2)
%#codegen

%    This function was generated by the Symbolic Math Toolbox version 8.7.
%    01-Jun-2022 14:38:05

G = [(g.*(L_2x.*m2.*cos(q1+q2)+L_1x.*m1.*cos(q1)+L_1x.*m2.*cos(q1).*2.0))./2.0;(L_2x.*g.*m2.*cos(q1+q2))./2.0];

== matlab function sim_2_twolink_joint_control_real/Controller/Inverse Dynamics control /MCKGQ ==
  data: L_1x input; M output; L_1y input; L_2x input; L_2y input; b1 input; b2 input; g input; m1 input; m2 input; q1 input; q2 input; q1_D input; q2_D input; tau1 input; tau2 input; C output; K output; G output; Q output
function [M,C,K,G,Q] = MCKGQ(L_1x,L_1y,L_2x,L_2y,b1,b2,g,m1,m2,q1,q2,q1_D,q2_D,tau1,tau2)
%#codegen

%    This function was generated by the Symbolic Math Toolbox version 8.7.
%    30-May-2022 13:59:37

M = reshape([(L_1x.^2.*m1)./3.0+L_1x.^2.*m2+(L_1y.^2.*m1)./1.2e+1+(L_2x.^2.*m2)./4.0+L_1x.*L_2x.*m2.*cos(q2),(L_2x.*m2.*(L_2x+L_1x.*cos(q2).*2.0))./4.0,(L_2x.*m2.*(L_2x+L_1x.*cos(q2).*2.0))./4.0,(m2.*(L_2x.^2.*4.0+L_2y.^2))./1.2e+1],[2,2]);
if nargout > 1
    C = reshape([-L_1x.*L_2x.*m2.*q2_D.*sin(q2),(L_1x.*L_2x.*m2.*q1_D.*sin(q2))./2.0,L_1x.*L_2x.*m2.*q2_D.*sin(q2).*(-1.0./2.0),0.0],[2,2]);
end
if nargout > 2
    K = reshape([0.0,0.0,0.0,0.0],[2,2]);
end
if nargout > 3
    G = [(g.*(L_2x.*m2.*cos(q1+q2)+L_1x.*m1.*cos(q1)+L_1x.*m2.*cos(q1).*2.0))./2.0;(L_2x.*g.*m2.*cos(q1+q2))./2.0];
end
if nargout > 4
    Q = [tau1-b1.*q1_D;tau2-b2.*q2_D];
end
